simulink model "pitch_angle_controller_variable_throttle"  (R2024b)
settings: Solver=ode1  StartTime=0.0  StopTime=120  FixedStep=0.1  RelTol=1e-3
values from neighbouring files (symbols this model uses):
  theta_0 = deg2rad(90)    [main.m]
  theta_ref = a0 + a1 * t + a2 * t.^2 + a3 * t.^3    [main.m]
libraries: simulink_extras x4, slpidlib x1
settings Model: Creator=jonathanvanzyl  LastModifiedBy=jonathanvanzyl

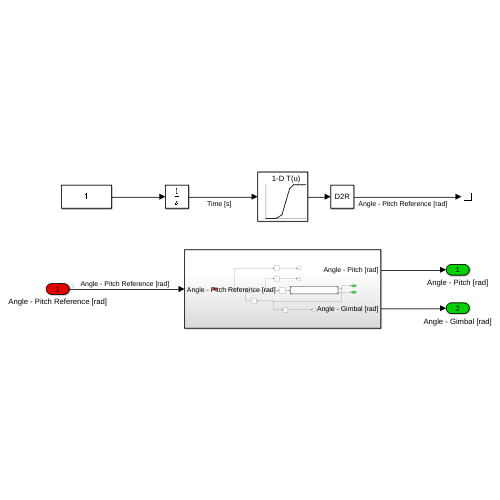
[thumbnail: Simulink's stored preview of the top-level diagram]
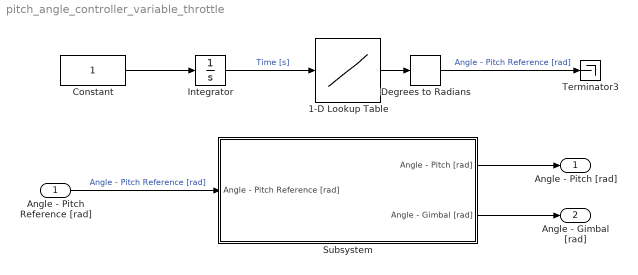
== system pitch_angle_controller_variable_throttle ==
  Angle - Pitch Reference [rad] : Inport
  1-D Lookup Table : Lookup_n-D  NumberOfTableDimensions=1  BreakpointsForDimension1=t  Table=theta_ref  InternalRulePriority=Speed  RndMeth=Simplest
  Constant : Constant
  Degrees to Radians : simulink_extras/Transformations/Degrees to Radians
  Integrator : Integrator
  Subsystem : Subsystem
  Terminator3 : Terminator
  Angle - Pitch [rad] : Outport
  Angle - Gimbal [rad] : Outport  Port=2
  wires:
  1-D Lookup Table/1 -> Degrees to Radians/1
  Integrator/1 -> 1-D Lookup Table/1  "Time [s]"
  Constant/1 -> Integrator/1
  Degrees to Radians/1 -> Terminator3/1  "Angle - Pitch Reference [rad]"
  Angle - Pitch Reference [rad]/1 -> Subsystem/1(Angle - Pitch Reference [rad])  "Angle - Pitch Reference [rad]"
  Subsystem/1(Angle - Pitch [rad]) -> Angle - Pitch [rad]/1
  Subsystem/2(Angle - Gimbal [rad]) -> Angle - Gimbal [rad]/1

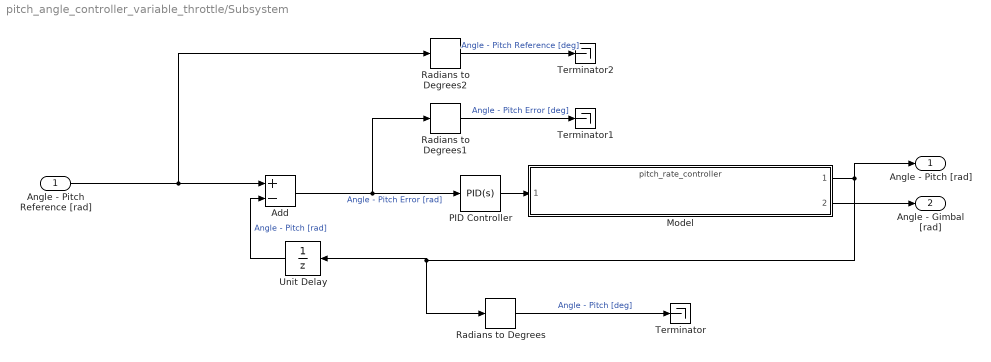
== system pitch_angle_controller_variable_throttle/Subsystem ==
  Angle - Pitch Reference [rad] : Inport
  Add : Sum  Inputs=+-
  Model : ModelReference  ModelNameDialog=pitch_rate_controller  SimulationMode=Normal  ModelReferenceVersion=1.8
  PID Controller : slpidlib/PID Controller  Controller=PID  Form=Parallel  TimeDomain=Continuous-time  UseExternalTs=off  SampleTime=-1  IntegratorMethod=Forward Euler  FilterMethod=Forward Euler  ControllerParametersSource=internal  P=0.5  I=0  UseKiTs=off  D=0  UseExternalDerivativeSource=off  N=100  UseFilter=on  TunerSelectOption=Transfer Function Based (PID Tuner App)  InitialConditionSource=internal  InitialConditionForIntegrator=0  InitialConditionForFilter=0  DifferentiatorICPrevScaledInput=0  ExternalReset=none  TrackingMode=off  Kt=1  LimitOutput=off  SatLimitsSource=internal  UpperSaturationLimit=inf  LowerSaturationLimit=-inf  LinearizeAsGain=on  AntiWindupMode=none  Kb=1  LimitIntegrator=off  UpperIntegratorSaturationLimit=inf  LowerIntegratorSaturationLimit=-inf  POutMin=[]  POutMax=[]  IOutMin=[]  IOutMax=[]  DOutMin=[]  DOutMax=[]  NOutMin=[]  NOutMax=[]  SumOutMin=[]  SumOutMax=[]  SaturationOutMin=[]  SaturationOutMax=[]  PParamMin=[]  PParamMax=[]  IParamMin=[]  IParamMax=[]  DParamMin=[]  DParamMax=[]  NParamMin=[]  NParamMax=[]  KbParamMin=[]  KbParamMax=[]  KtParamMin=[]  KtParamMax=[]  KbOutMin=[]  KbOutMax=[]  KtOutMin=[]  KtOutMax=[]  IntegratorOutMin=[]  IntegratorOutMax=[]  FilterOutMin=[]  FilterOutMax=[]  SumI1OutMin=[]  SumI1OutMax=[]  SumI2OutMin=[]  SumI2OutMax=[]  SumI3OutMin=[]  SumI3OutMax=[]  SumI4OutMin=[]  SumI4OutMax=[]  SumDOutMin=[]  SumDOutMax=[]  DifferentiatorOutMin=[]  DifferentiatorOutMax=[]  FilterDiffOutCoefMin=[]  FilterDiffOutCoefMax=[]  ReciprocalOutMin=[]  ReciprocalOutMax=[]  SumDenOutMin=[]  SumDenOutMax=[]  SumNumOutMin=[]  SumNumOutMax=[]  DivideOutMin=[]  DivideOutMax=[]  UdiffTsProdOutMin=[]  UdiffTsProdOutMax=[]  NTsProdOutMin=[]  NTsProdOutMax=[]  UintegralTsProdOutMin=[]  UintegralTsProdOutMax=[]  UngainTsProdOutMin=[]  UngainTsProdOutMax=[]  ClampingZeroOutDataTypeStr=Inherit: Inherit via back propagation  ClampingZeroOutMin=[]  ClampingZeroOutMax=[]  FilterDenConstantOutDataTypeStr=Inherit: Inherit via back propagation  FilterDenConstantOutMin=[]  FilterDenConstantOutMax=[]  PCopyOutDataTypeStr=Inherit: Inherit via back propagation  PCopyOutMin=[]  PCopyOutMax=[]  NCopyOutDataTypeStr=Inherit: Inherit via back propagation  NCopyOutMin=[]  NCopyOutMax=[]  IntegratorContinuousStateAttributes=''  IntegratorStateMustResolveToSignalObject=off  IntegratorRTWStateStorageClass=Auto  FilterContinuousStateAttributes=''  FilterStateMustResolveToSignalObject=off  FilterRTWStateStorageClass=Auto  ParallelPVariant=InternalParameters  IdealPVariant=Disabled  IVariant=InternalParameters  DVariant=InternalParameters  IntegratorVariant=Continuous  SatVariant=Disabled  AWVariant=Passthrough  PCopyVariant=Disabled  TRVariant=Disabled  FdbkBlocksVariant=Forward  IdealPFdbkVariant=Disabled  SatFdbkVariant=Disabled  DerivativeFilterVariant=ContFilter  NVariant=InternalParameters  NCopyVariant=Disabled  FilterICVariant=InternalICsFilter  IntegratorICVariant=InternalICs  ExternalResetVariant=Disabled  TRSumVariant=Passthrough  SumFdbkVariant=Disabled  SumVariant=Sum_PID  TsampFilterVariant=InternalTs  TsampNgainVariant=Passthrough  TsampIntegralVariant=Disabled_SignalSpec  ExternalSaturationOutDataTypeStr=Inherit: Same as second input  DerivativeSourceVariant=ErrorSignal  PreIntVariant=InternalPreInt
  Radians to Degrees : simulink_extras/Transformations/Radians to Degrees
  Radians to Degrees1 : simulink_extras/Transformations/Radians to Degrees
  Radians to Degrees2 : simulink_extras/Transformations/Radians to Degrees
  Terminator : Terminator
  Terminator1 : Terminator
  Terminator2 : Terminator
  Unit Delay : UnitDelay  InitialCondition=theta_0  SampleTime=-1  HasFrameUpgradeWarning=on
  Angle - Pitch [rad] : Outport
  Angle - Gimbal [rad] : Outport  Port=2
  wires:
  Radians to Degrees2/1 -> Terminator2/1  "Angle - Pitch Reference [deg]"
  Radians to Degrees/1 -> Terminator/1  "Angle - Pitch [deg]"
  Add/1 -> Radians to Degrees1/1, PID Controller/1  "Angle - Pitch Error [rad]"
  Unit Delay/1 -> Add/2  "Angle - Pitch [rad]"
  Model/2 -> Angle - Gimbal [rad]/1
  Angle - Pitch Reference [rad]/1 -> Radians to Degrees2/1, Add/1
  PID Controller/1 -> Model/1
  Radians to Degrees1/1 -> Terminator1/1  "Angle - Pitch Error [deg]"
  Model/1 -> Angle - Pitch [rad]/1, Radians to Degrees/1, Unit Delay/1
